simulink model "INTERLOCK_DELAY"  (R2016a)
settings: Solver=FixedStepDiscrete  StartTime=0.0  StopTime=10.0  RelTol=1e-3
values from neighbouring files (symbols this model uses):
  INVERSE_BOTTOMSWITCH = 0    [Init_InterLock.m]
undefined symbols (not defined in the file or in its folder): sigbuilder_block
libraries: simulink x12
settings Model: Creator=zedboard  LastModifiedBy=Wendel
settings OptimizationCC: BlockReduction=off  ConditionallyExecuteInputs=off  DefaultParameterBehavior=Inlined
settings DebuggingCC: AlgebraicLoopMsg=error
settings HardwareCC: ProdBitPerPointer=32  ProdLargestAtomicFloat=None  ProdIntDivRoundTo=Undefined  ProdEndianess=Unspecified  ProdWordSize=32  ProdHWDeviceType=ASIC/FPGA->ASIC/FPGA  ProdEqTarget=off

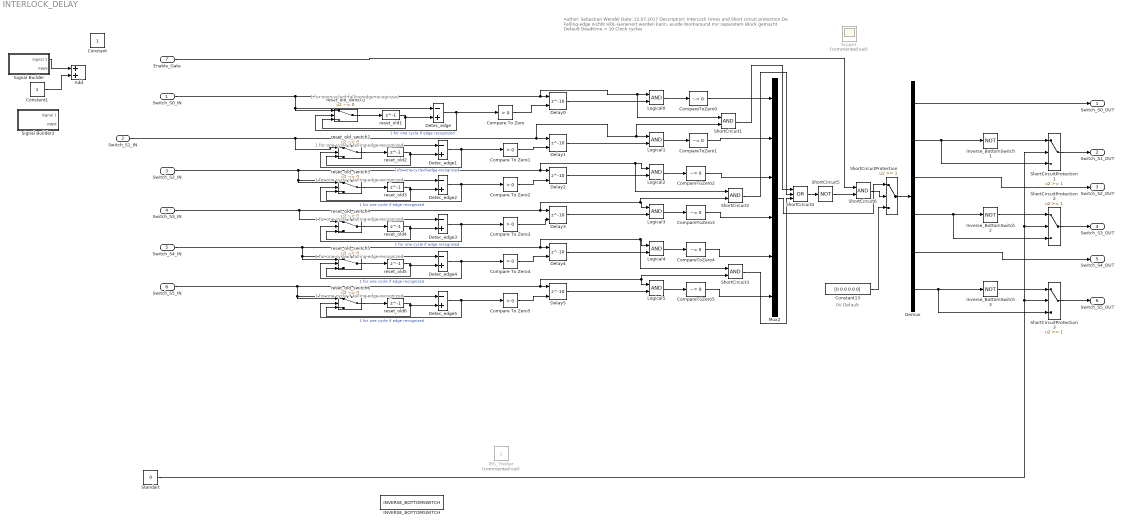
== system INTERLOCK_DELAY ==
  note: Author: Sebastian Wendel
      | Date: 22.07.2017
      | Description:
      | InterLock times and Short circuit protection
      | Da Falling-edge nichht HDL-Generiert werden kann, wurde Workaround mir separatem Block gemacht
      | Default Deadtime = 10 Clock cycles
  note: 0V Default
  note: 1 for one cycle if falling edge recognized
  note: 1 for one cycle if falling edge recognized
  note: 1 for one cycle if falling edge recognized
  note: 1 for one cycle if falling edge recognized
  note: 1 for one cycle if falling edge recognized
  note: 1 for one cycle if falling edge recognized
  Switch_S0_IN : Inport  OutDataTypeStr=boolean
  Switch_S1_IN : Inport  Port=2  OutDataTypeStr=boolean
  Switch_S2_IN : Inport  Port=3  OutDataTypeStr=boolean
  Switch_S3_IN : Inport  Port=4  OutDataTypeStr=boolean
  Switch_S4_IN : Inport  Port=5  OutDataTypeStr=boolean
  Switch_S5_IN : Inport  Port=6  OutDataTypeStr=boolean
  Enable_Gate : Inport  Port=7  OutDataTypeStr=boolean
  Add : Sum
  Compare To Zero{,1..5} (6 alike) : simulink/Logic and Bit Operations/Compare To Zero  relop=>  OutDataTypeStr=boolean
  CompareToZero{0..5} (6 alike) : simulink/Logic and Bit Operations/Compare To Zero  relop=~=  OutDataTypeStr=boolean
  Constant : Constant
  Constant1 : Constant
  Constant13 : Constant  Value=[0 0 0 0 0 0]  OutDataTypeStr=boolean  SampleTime=-1
  Delay{0..5} (6 alike) : Delay  DelayLength=10  InitialCondition=0  ExternalReset=Level
      settings: InputPortMap=u0,r5
  Demux : Demux  Outputs=6
  Detec_edge{,1..5} (6 alike) : Sum  Inputs=-+  AccumDataTypeStr=int8  OutDataTypeStr=int8
  INVERSE_BOTTOMSWITCH : Constant  Value=INVERSE_BOTTOMSWITCH  OutDataTypeStr=boolean  SampleTime=-1
  IRS_Treiber : Constant  Commented=on
  Inverse_BottomSwitch1 : Logic  Operator=NOT  Inputs=3  AllPortsSameDT=off  OutDataTypeStr=boolean
  Inverse_BottomSwitch2 : Logic  Operator=NOT  Inputs=3  AllPortsSameDT=off  OutDataTypeStr=boolean
  Inverse_BottomSwitch3 : Logic  Operator=NOT  Inputs=3  AllPortsSameDT=off  OutDataTypeStr=boolean
  Logical{0..5} (6 alike) : Logic  AllPortsSameDT=off  OutDataTypeStr=boolean
  Mux2 : Mux  Inputs=6
  Scope1 : Scope  Commented=on  NumInputPorts=3
  ShortCircuit{1..3,6} (4 alike) : Logic  AllPortsSameDT=off  OutDataTypeStr=boolean
  ShortCircuit4 : Logic  Operator=OR  Inputs=3  AllPortsSameDT=off  OutDataTypeStr=boolean
  ShortCircuit5 : Logic  Operator=NOT  Inputs=3  AllPortsSameDT=off  OutDataTypeStr=boolean
  ShortCircuitProtection{,1..3} (4 alike) : Switch  Threshold=1
  Signal Builder : Subsystem  Tag=STV Subsys  LoadFcn=sigbuilder_block('load');  StartFcn=sigbuilder_block('start');  StopFcn=sigbuilder_block('stop');  ClipboardFcn=sigbuilder_block('clipboard');  mask(Sigbuilder block){}
      mask help: Simulink:masks:SigbuilderBlock_MD
      mask init:
      | if ~strcmp(get_param(bdroot(gcbh),'SimulationStatus'),'stopped') tuvar = sigbuilder_block('maskInit'); end
      settings: CopyFcn=sigbuilder_block('copy');  DeleteFcn=sigbuilder_block('delete');  ModelCloseFcn=sigbuilder_block('modelClose');  PreSaveFcn=sigbuilder_block('preSave');  PauseFcn=sigbuilder_block('pause');  ContinueFcn=sigbuilder_block('continue');  NameChangeFcn=sigbuilder_block('namechange');  OpenFcn=sigbuilder_block('open',[5.4 30 1141.2 522.6 ]);  CloseFcn=sigbuilder_block('close');
      mask Display: plot(0, 0, 100, 100,[2, 2, 32, 32, 2], [68, 8, 8, 68, 68],[32, 2], [38, 38], [32, 19, 2],[53, 60, 44], [32, 17, 17, 2],[16, 16, 31, 31]);txt = getActiveGroup(gcbh);text(2, 100, txt,'verticalAlignment', 'top');
  Signal Builder2 : Subsystem  Tag=STV Subsys  LoadFcn=sigbuilder_block('load');  StartFcn=sigbuilder_block('start');  StopFcn=sigbuilder_block('stop');  ClipboardFcn=sigbuilder_block('clipboard');  mask(Sigbuilder block){}
      mask help: Simulink:masks:SigbuilderBlock_MD
      mask init:
      | if ~strcmp(get_param(bdroot(gcbh),'SimulationStatus'),'stopped') tuvar = sigbuilder_block('maskInit'); end
      settings: CopyFcn=sigbuilder_block('copy');  DeleteFcn=sigbuilder_block('delete');  ModelCloseFcn=sigbuilder_block('modelClose');  PreSaveFcn=sigbuilder_block('preSave');  PauseFcn=sigbuilder_block('pause');  ContinueFcn=sigbuilder_block('continue');  NameChangeFcn=sigbuilder_block('namechange');  OpenFcn=sigbuilder_block('open',[0 30 1152 561.6 ]);  CloseFcn=sigbuilder_block('close');
      mask Display: plot(0, 0, 100, 100,[2, 2, 32, 32, 2], [68, 8, 8, 68, 68],[32, 2], [38, 38], [32, 19, 2],[53, 60, 44], [32, 17, 17, 2],[16, 16, 31, 31]);txt = getActiveGroup(gcbh);text(2, 100, txt,'verticalAlignment', 'top');
  Standart : Constant  Value=0
  reset_old{1..6} (6 alike) : Delay  DelayLength=1
  reset_old_switch{1..6} (6 alike) : Switch  Criteria=u2 ~= 0
  Switch_S0_OUT : Outport
  Switch_S1_OUT : Outport  Port=2
  Switch_S2_OUT : Outport  Port=3
  Switch_S3_OUT : Outport  Port=4
  Switch_S4_OUT : Outport  Port=5
  Switch_S5_OUT : Outport  Port=6
  wires:
  Delay0/1 -> Logical0/2
  Logical0/1 -> CompareToZero0/1
  CompareToZero0/1 -> Mux2/1
  Enable_Gate/1 -> ShortCircuit6/1
  Delay1/1 -> Logical1/2
  Logical1/1 -> CompareToZero1/1
  CompareToZero1/1 -> Mux2/2
  Delay2/1 -> Logical2/2
  Logical2/1 -> CompareToZero2/1
  CompareToZero2/1 -> Mux2/3
  Delay3/1 -> Logical3/2
  Logical3/1 -> CompareToZero3/1
  CompareToZero3/1 -> Mux2/4
  Delay4/1 -> Logical4/2
  Logical4/1 -> CompareToZero4/1
  CompareToZero4/1 -> Mux2/5
  Delay5/1 -> Logical5/2
  Logical5/1 -> CompareToZero5/1
  CompareToZero5/1 -> Mux2/6
  Mux2/1 -> ShortCircuitProtection/1
  Constant13/1 -> ShortCircuitProtection/3
  ShortCircuitProtection/1 -> Demux/1
  Demux/2 -> ShortCircuitProtection1/3, Inverse_BottomSwitch1/1
  Demux/3 -> Switch_S2_OUT/1
  Demux/5 -> Switch_S4_OUT/1
  ShortCircuit4/1 -> ShortCircuit5/1
  ShortCircuit1/1 -> ShortCircuit4/1
  ShortCircuit2/1 -> ShortCircuit4/2
  ShortCircuit3/1 -> ShortCircuit4/3
  ShortCircuit6/1 -> ShortCircuitProtection/2
  ShortCircuit5/1 -> ShortCircuit6/2
  Inverse_BottomSwitch1/1 -> ShortCircuitProtection1/1
  ShortCircuitProtection1/1 -> Switch_S1_OUT/1
  Demux/4 -> ShortCircuitProtection2/3, Inverse_BottomSwitch2/1
  Inverse_BottomSwitch2/1 -> ShortCircuitProtection2/1
  ShortCircuitProtection2/1 -> Switch_S3_OUT/1
  Demux/6 -> Inverse_BottomSwitch3/1, ShortCircuitProtection3/3
  Inverse_BottomSwitch3/1 -> ShortCircuitProtection3/1
  ShortCircuitProtection3/1 -> Switch_S5_OUT/1
  Standart/1 -> ShortCircuitProtection1/2, ShortCircuitProtection2/2, ShortCircuitProtection3/2
  Demux/1 -> Switch_S0_OUT/1
  Compare To Zero5/1 -> Delay5/2
  Compare To Zero4/1 -> Delay4/2
  Compare To Zero2/1 -> Delay2/2
  Compare To Zero1/1 -> Delay1/2
  Compare To Zero/1 -> Delay0/2
  Compare To Zero3/1 -> Delay3/2
  reset_old_switch1/1 -> reset_old1/1
  reset_old1/1 -> reset_old_switch1/3, Detec_edge/2
  Detec_edge/1 -> Compare To Zero/1, reset_old_switch1/2  "1 for one cycle if edge recognized"
  reset_old_switch2/1 -> reset_old2/1
  Switch_S1_IN/1 -> Detec_edge1/1, reset_old_switch2/1, ShortCircuit1/2, Logical1/1, Delay1/1
  reset_old2/1 -> reset_old_switch2/3, Detec_edge1/2
  Detec_edge1/1 -> Compare To Zero1/1, reset_old_switch2/2  "1 for one cycle if edge recognized"
  reset_old_switch3/1 -> reset_old3/1
  Switch_S2_IN/1 -> ShortCircuit2/1, Logical2/1, Delay2/1, reset_old_switch3/1, Detec_edge2/1
  reset_old3/1 -> reset_old_switch3/3, Detec_edge2/2
  Detec_edge2/1 -> Compare To Zero2/1, reset_old_switch3/2  "1 for one cycle if edge recognized"
  reset_old_switch4/1 -> reset_old4/1
  Switch_S3_IN/1 -> ShortCircuit2/2, Logical3/1, Delay3/1, reset_old_switch4/1, Detec_edge3/1
  reset_old4/1 -> reset_old_switch4/3, Detec_edge3/2
  Detec_edge3/1 -> Compare To Zero3/1, reset_old_switch4/2  "1 for one cycle if edge recognized"
  reset_old_switch5/1 -> reset_old5/1
  Switch_S4_IN/1 -> Delay4/1, ShortCircuit3/1, Logical4/1, reset_old_switch5/1, Detec_edge4/1
  reset_old5/1 -> reset_old_switch5/3, Detec_edge4/2
  Detec_edge4/1 -> Compare To Zero4/1, reset_old_switch5/2  "1 for one cycle if edge recognized"
  reset_old_switch6/1 -> reset_old6/1
  Switch_S5_IN/1 -> Delay5/1, ShortCircuit3/2, Logical5/1, reset_old_switch6/1, Detec_edge5/1
  reset_old6/1 -> reset_old_switch6/3, Detec_edge5/2
  Detec_edge5/1 -> Compare To Zero5/1, reset_old_switch6/2  "1 for one cycle if edge recognized"
  Constant1/1 -> Add/2
  Signal Builder/1(Signal 1) -> Add/1
  Switch_S0_IN/1 -> Delay0/1, ShortCircuit1/1, Logical0/1, reset_old_switch1/1, Detec_edge/1

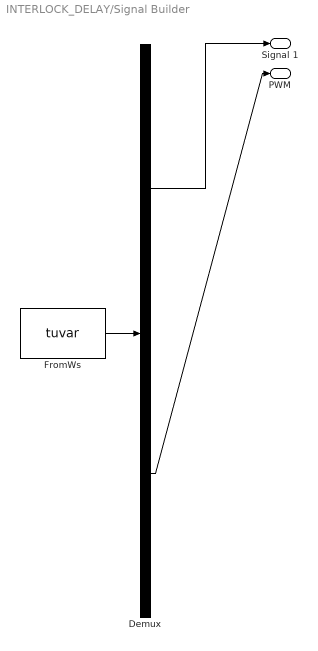
== system INTERLOCK_DELAY/Signal Builder ==
  Demux : Demux  Tag=STV Demux  Outputs=2
  FromWs : FromWorkspace  Tag=STV FromWs  VariableName=tuvar  SampleTime=0
      SigBuilderData=|
      | common.afterFinalStr = 'Extrapolate'
      | common.sampleTime = 0
      | dataSet.timeRange = [0 10]
      | dataSet.name = 'Group 1'
      | sbobj.Groups.Name = 'Group 1'
      | sbobj.Groups.Signals(1).Name = 'Signal 1'
      | sbobj.Groups.Signals(1).XData = [0 1.02 1.02 6 6 10]
      | sbobj.Groups.Signals(1).YData = [0 0 1 1 0 0]
      | sbobj.Groups.Signals(2).Name = 'PWM'
      | sbobj.Groups.Signals(2).XData = [0 0.01 0.01 0.02 0.02 0.03 0.03 0.04 0.04 0.05 0.05 0.06 ... (1997 elements, 1x1997)]
      | sbobj.Groups.Signals(2).YData = [-1 -1 0 0 -1 -1 0 0 -1 -1 0 0 ... (1997 elements, 1x1997)]
  Signal 1 : Outport  Tag=STV Outport
  PWM : Outport  Tag=STV Outport  Port=2
  wires:
  Demux/1 -> Signal 1/1
  FromWs/1 -> Demux/1
  Demux/2 -> PWM/1

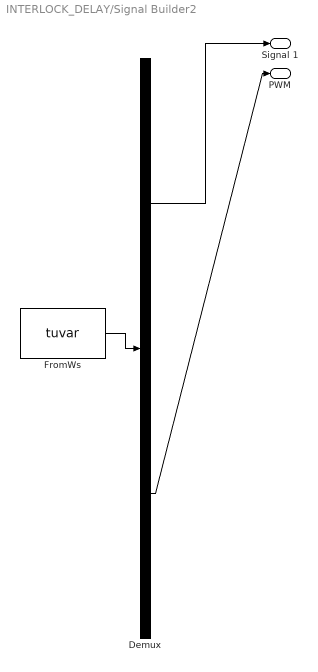
== system INTERLOCK_DELAY/Signal Builder2 ==
  Demux : Demux  Tag=STV Demux  Outputs=2
  FromWs : FromWorkspace  Tag=STV FromWs  VariableName=tuvar  SampleTime=0
      SigBuilderData=|
      | common.afterFinalStr = 'Extrapolate'
      | common.sampleTime = 0
      | dataSet.timeRange = [0 10]
      | dataSet.name = 'Group 1'
      | sbobj.Groups.Name = 'Group 1'
      | sbobj.Groups.Signals(1).Name = 'Signal 1'
      | sbobj.Groups.Signals(1).XData = [0 1.9 1.9 8 8 10]
      | sbobj.Groups.Signals(1).YData = [0 0 1 1 0 0]
      | sbobj.Groups.Signals(2).Name = 'PWM'
      | sbobj.Groups.Signals(2).XData = [0 0.01 0.01 0.02 0.02 0.03 0.03 0.04 0.04 0.05 0.05 0.06 ... (2000 elements, 1x2000)]
      | sbobj.Groups.Signals(2).YData = [1 1 0 0 1 1 0 0 1 1 0 0 ... (2000 elements, 1x2000)]
  Signal 1 : Outport  Tag=STV Outport
  PWM : Outport  Tag=STV Outport  Port=2
  wires:
  Demux/1 -> Signal 1/1
  FromWs/1 -> Demux/1
  Demux/2 -> PWM/1
